simulink model "pend"  (R2016b)
settings: Solver=VariableStepAuto  StartTime=0.0  StopTime=10.0  RelTol=1e-3
values from neighbouring files (symbols this model uses):
  g = 9.81    [pend.m]
  l = 0.5    [pend.m]
  m = 0.1    [pend.m]
  mc = 1    [pend.m]
  x1_0 = 1    [pend.m]
  x2_0 = 2    [pend.m]
libraries: fuzblock x1
settings Model: Creator=Mee  LastModifiedBy=Mee

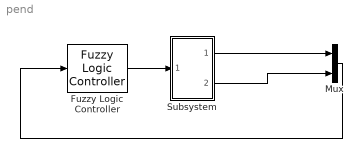
== system pend ==
  Fuzzy Logic Controller : fuzblock/Fuzzy Logic  Controller  fis='PANDULUM.fis'
  Mux : Mux  Inputs=2
  Subsystem : Subsystem
  wires:
  Fuzzy Logic Controller/1 -> Subsystem/1(In1)
  Subsystem/1(Out1) -> Mux/1
  Subsystem/2(Out2) -> Mux/2
  Mux/1 -> Fuzzy Logic Controller/1

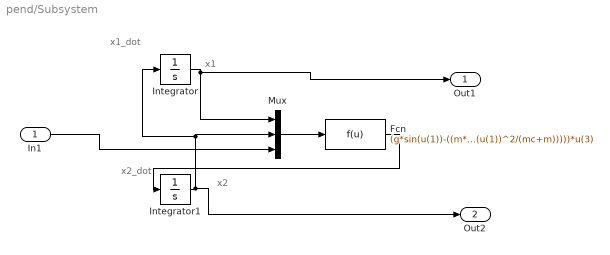
== system pend/Subsystem ==
  note: x2_dot
  note: x1_dot
  note: x2
  note: x1
  In1 : Inport
  Fcn : Fcn  Expr=(g*sin(u(1))-((m*l*u(2)^2*cos(u(1))*sin(u(1))/(mc+m))))/(l*(4/3-(m*cos(u(1))^2/(mc+m))))+(cos(u(1))/(mc+m))/((l*(4/3-(m*cos(u(1))^2/(mc+m)))))*u(3)
  Integrator : Integrator  InitialCondition=x1_0
  Integrator1 : Integrator  InitialCondition=x2_0
  Mux : Mux  Inputs=3
  Out1 : Outport
  Out2 : Outport  Port=2
  wires:
  In1/1 -> Mux/3
  Mux/1 -> Fcn/1
  Integrator/1 -> Out1/1, Mux/1
  Fcn/1 -> Integrator1/1
  Integrator1/1 -> Out2/1, Mux/2, Integrator/1
